simulink model "lab4pt3SFI"  (R2012b)
settings: Solver=ode1  StartTime=0.0  StopTime=10  FixedStep=0.002  RelTol=1e-3
values from neighbouring files (symbols this model uses):
  g = 9.78    [lab4prelab.m]
  l = 0.303    [lab4prelab.m]
  M = 0.455    [lab4prelab.m]
  m = 0.210    (= 0.21)    [lab4prelab.m]
undefined symbols (not defined in the file or in its folder): theta_0, theta_dot_0, x_0, x_dot_0
settings Model: ExtModeTrigDuration=5000  Creator=vukovic8  LastModifiedBy=vukovic8
settings SolverCC: PositivePriorityOrder=on
settings RTWCC: SystemTargetFile=quarc_win64.tlc  TemplateMakefile=quarc_default_tmf  Description=QUARC Win64 Target  ProcessScript=quarc_win64_make_rtw_hook
settings STFCustomTargetCC: TargetPreCompLibLocation=C:\PROGRA~3\QUARC\lib\2012b\win64\release  CodeReplacementLibrary=ANSI_C  GeneratePreprocessorConditionals=Disable all  CombineOutputUpdateFcns=on  GRTInterface=off  SystemTargetFile=quarc_win64.tlc
settings GRTTargetCC: TargetPreCompLibLocation=C:\PROGRA~3\QUARC\lib\2012b\win64\release  ParMdlRefBuildCompliant=off  CompOptLevelCompliant=off  ConcurrentExecutionCompliant=off  MatFileLogging=off  ExtMode=on  ExtModeMexFile=quarc_comm

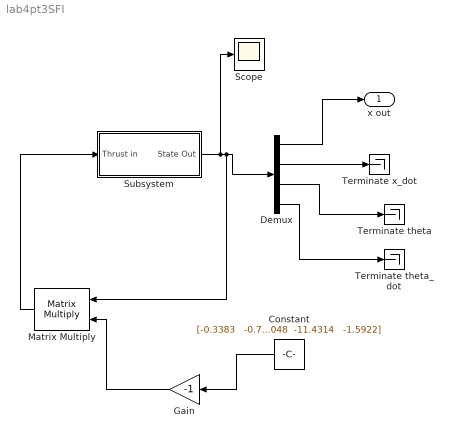
== system lab4pt3SFI ==
  Constant : Constant  Value="[-0.3383   -0.7048  -11.4314   -1.5922]"
  Demux : Demux
  Gain : Gain  Gain=-1
  Matrix Multiply : Product  Multiplication=Matrix(*)
  Scope : Scope
  Subsystem : Subsystem
  Terminate theta : Terminator
  Terminate theta_dot : Terminator
  Terminate x_dot : Terminator
  x out : Outport
  wires:
  Demux/1 -> x out/1
  Demux/2 -> Terminate x_dot/1
  Demux/3 -> Terminate theta/1
  Demux/4 -> Terminate theta_dot/1
  Subsystem/1(State Out) -> Scope/1, Matrix Multiply/1, Demux/1
  Constant/1 -> Gain/1
  Gain/1 -> Matrix Multiply/2
  Matrix Multiply/1 -> Subsystem/1(Thrust in)

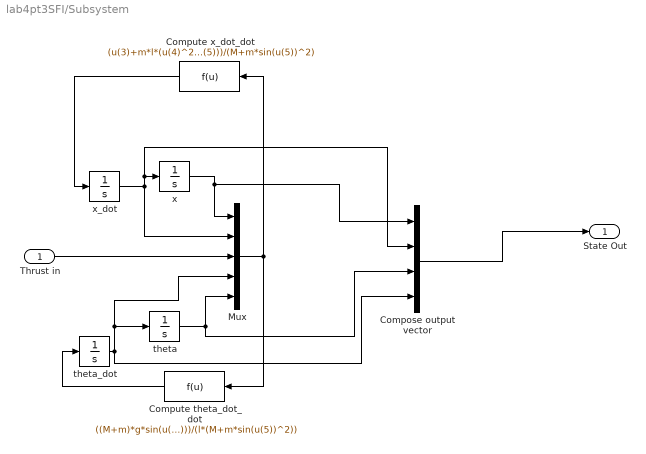
== system lab4pt3SFI/Subsystem ==
  Thrust in : Inport
  Compose output vector : Mux
  Compute theta_dot_dot : Fcn  Expr=((M+m)*g*sin(u(5))-u(3)*cos(u(5))-m*l*(u(4))^2*sin(u(5))*cos(u(5)))/(l*(M+m*sin(u(5))^2))
  Compute x_dot_dot : Fcn  Expr=(u(3)+m*l*(u(4)^2)*sin(u(5)) - m*g*cos(u(5))*sin(u(5)))/(M+m*sin(u(5))^2)
  Mux : Mux  Inputs=5
  theta : Integrator  InitialCondition=theta_0
  theta_dot : Integrator  InitialCondition=theta_dot_0
  x : Integrator  InitialCondition=x_0
  x_dot : Integrator  InitialCondition=x_dot_0
  State Out : Outport
  wires:
  Thrust in/1 -> Mux/3
  Mux/1 -> Compute x_dot_dot/1, Compute theta_dot_dot/1
  Compute theta_dot_dot/1 -> theta_dot/1
  theta_dot/1 -> theta/1, Mux/4, Compose output vector/4
  theta/1 -> Mux/5, Compose output vector/3
  Compute x_dot_dot/1 -> x_dot/1
  x_dot/1 -> Compose output vector/2, x/1, Mux/2
  x/1 -> Compose output vector/1, Mux/1
  Compose output vector/1 -> State Out/1
